simulink model "VDCHyd2020a"  (R2020a)
settings: Solver=daessc  StartTime=0.0  StopTime=simulationEndTime  FixedStep=0.001  RelTol=1e-2
values from neighbouring files (symbols this model uses):
  Bc1_V = [0;0;0;0;0;0]    [initializeSimulationGP.m]
  filtDV = init2ndOrderLowPassFilter(35*2*pi,1,controller.dT)    [initializeLowPassFilters.m]
  filtEnc = init2ndOrderLowPassFilter(35*2*pi,1,controller.dT)    [initializeLowPassFilters.m]
undefined symbols (not defined in the file or in its folder): aux, B11_r_B11Tc1, B11_V, B11_Vr, B11Ftot_r, B12_r_B12Tc2, B12_Rot_Tc2, B12_U_Tc2, B12_V, B12_Vr, B12Ftot_r, B31_r_B31B41, B31_V, B31_Vr, B31FTot_r, B32_r_B32B42, B32_Rot_B42, B32_U_B42, B32_V, B32_Vr, B32FTot_r, B41_r_B41Tc1, B41_V, B41_Vr, B41FTot_r, B42_r_B42Tc2, B42_Rot_Tc2, B42_U_Tc2, B42_V, B42_Vr, B42FTot_r, B52_r_B52P32, B52_Rot_P32, B52_U_P32, B52_V, B52_Vr, B52Ftot_r, Bc1_r_Bc1B11, Bc1_r_Bc1B31, Bc1_Vr, Bc1FTot_r, Bc2_r_Bc2B12, Bc2_r_Bc2B32, Bc2_Rot_B12, Bc2_Rot_B32, Bc2_U_B12, Bc2_U_B32, Bc2_V, Bc2_Vr, Bc2Tot_r, controller, cyl1, cyl2, cylT2, D22_V, D22_Vr, D22Fr, DiscIntNeverNeededParam, dq1, dq11 ... (+125)
libraries: sm_lib x34, nesl_utility x15, simulink x11, dspinverses x1
(part 7 of 12)

== system VDCHyd2020a/sbVDCController/sbFormTotalRequiredForces/sbTotalRequiredForcesPS2/sbProjectionFunctionB52 ==
  note: dP_{B_{52}} / dt = \rho_{B_{52}} s_{B_{52}} \kappa
  sB52 : Inport  PortDimensions=13
  updateActive : Inport  Port=2
  updateReset : Inport  Port=3  PortDimensions=1
  Constant : Constant  Value=update.thetaB52rNominal
  Switch : Switch  Criteria=u2 > Threshold
  discreteIntegratorB52 : DiscreteIntegrator  IntegratorMethod=Integration: Trapezoidal  gainval=update.rhoB52  ExternalReset=level  InitialConditionSource=external  InitialCondition=update.thetaB52rNominal  SampleTime=controller.dT  LimitOutput=on  UpperSaturationLimit=update.thetaB52rUpperBound  LowerSaturationLimit=update.thetaB52rLowerBound  ICPrevOutput=DiscIntNeverNeededParam  ICPrevScaledInput=DiscIntNeverNeededParam
  thetaB52r : Outport
  wires:
  sB52/1 -> discreteIntegratorB52/1  "sB52"
  updateActive/1 -> Switch/2  "updParams"
  Switch/1 -> thetaB52r/1  "thetaB52r"
  Constant/1 -> Switch/3, discreteIntegratorB52/3  "thetaB52rNominal"
  discreteIntegratorB52/1 -> Switch/1  "thetaB52rUpdated"
  updateReset/1 -> discreteIntegratorB52/2  "updateReset"

== system VDCHyd2020a/sbVDCController/sbFormTotalRequiredForces/sbTotalRequiredForcesPS2/sbProjectionFunctionP22 ==
  note: dP_{P_{22}} / dt = \rho_{P_{22}} s_{P_{22}} \kappa
  sP22 : Inport  PortDimensions=13
  updateActive : Inport  Port=2
  updateReset : Inport  Port=3  PortDimensions=1
  Constant : Constant  Value=update.thetaP22rNominal
  Switch : Switch  Criteria=u2 > Threshold
  discreteIntegratorP22 : DiscreteIntegrator  IntegratorMethod=Integration: Trapezoidal  gainval=update.rhoP22  ExternalReset=level  InitialConditionSource=external  InitialCondition=update.thetaP22rNominal  SampleTime=controller.dT  LimitOutput=on  UpperSaturationLimit=update.thetaP22rUpperBound  LowerSaturationLimit=update.thetaP22rLowerBound  ICPrevOutput=DiscIntNeverNeededParam  ICPrevScaledInput=DiscIntNeverNeededParam
  thetaP22r : Outport
  wires:
  updateReset/1 -> discreteIntegratorP22/2  "updateReset"
  discreteIntegratorP22/1 -> Switch/1  "thetaP22rUpdated"
  Constant/1 -> Switch/3, discreteIntegratorP22/3  "thetaP22rNominal"
  Switch/1 -> thetaP22r/1  "thetaP22r"
  updateActive/1 -> Switch/2  "updateActive"
  sP22/1 -> discreteIntegratorP22/1  "sP22"

== system VDCHyd2020a/sbVDCController/sbFormTotalRequiredForces/sbTotalRequiredForcesPS2/sbProjectionFunctionP32 ==
  note: dP_{P_{32}} / dt = \rho_{P_{32}} s_{P_{32}} \kappa
  sP32 : Inport  PortDimensions=13
  updateActive : Inport  Port=2
  updateReset : Inport  Port=3  PortDimensions=1
  Constant : Constant  Value=update.thetaP32rNominal
  Switch : Switch  Criteria=u2 > Threshold
  discreteIntegratorP32 : DiscreteIntegrator  IntegratorMethod=Integration: Trapezoidal  gainval=update.rhoP32  ExternalReset=level  InitialConditionSource=external  InitialCondition=update.thetaP32rNominal  SampleTime=controller.dT  LimitOutput=on  UpperSaturationLimit=update.thetaP32rUpperBound  LowerSaturationLimit=update.thetaP32rLowerBound  ICPrevOutput=DiscIntNeverNeededParam  ICPrevScaledInput=DiscIntNeverNeededParam
  thetaP32r : Outport
  wires:
  updateReset/1 -> discreteIntegratorP32/2  "updateReset"
  discreteIntegratorP32/1 -> Switch/1  "thetaP32rUpdate"
  Constant/1 -> Switch/3, discreteIntegratorP32/3  "thetaP32rNominal"
  Switch/1 -> thetaP32r/1  "thetaP32r"
  updateActive/1 -> Switch/2  "updateActive"
  sP32/1 -> discreteIntegratorP32/1  "sP32"

== system VDCHyd2020a/sbVDCController/sbFormTotalRequiredForces/sbTotalRequiredForcesRS1/sbFilteredVelocityDerivativeB11 ==
  u : Inport
  Demux : Demux  Outputs=6
  Mux : Mux  Inputs=6
  sbDiscreteDerivative1 : Subsystem
  sbDiscreteDerivative2 : Subsystem
  sbDiscreteDerivative3 : Subsystem
  sbDiscreteDerivative4 : Subsystem
  sbDiscreteDerivative5 : Subsystem
  sbDiscreteDerivative6 : Subsystem
  sbLowPassFilter1 : Subsystem
  sbLowPassFilter2 : Subsystem
  sbLowPassFilter3 : Subsystem
  sbLowPassFilter4 : Subsystem
  sbLowPassFilter5 : Subsystem
  sbLowPassFilter6 : Subsystem
  du : Outport
  wires:
  sbLowPassFilter5/1(dVFilt) -> Mux/5
  sbDiscreteDerivative4/1(du/dt) -> sbLowPassFilter4/1(dV)
  sbLowPassFilter4/1(dVFilt) -> Mux/4
  sbLowPassFilter3/1(dVFilt) -> Mux/3
  sbDiscreteDerivative3/1(du/dt) -> sbLowPassFilter3/1(dV)
  sbDiscreteDerivative2/1(du/dt) -> sbLowPassFilter2/1(dV)
  sbLowPassFilter6/1(dVFilt) -> Mux/6
  sbDiscreteDerivative6/1(du/dt) -> sbLowPassFilter6/1(dV)
  sbLowPassFilter1/1(dVFilt) -> Mux/1
  u/1 -> Demux/1
  Demux/2 -> sbDiscreteDerivative2/1(u)
  Demux/5 -> sbDiscreteDerivative5/1(u)
  sbDiscreteDerivative1/1(du/dt) -> sbLowPassFilter1/1(dV)
  Demux/6 -> sbDiscreteDerivative6/1(u)
  sbLowPassFilter2/1(dVFilt) -> Mux/2
  Demux/1 -> sbDiscreteDerivative1/1(u)
  Demux/4 -> sbDiscreteDerivative4/1(u)
  Mux/1 -> du/1
  sbDiscreteDerivative5/1(du/dt) -> sbLowPassFilter5/1(dV)
  Demux/3 -> sbDiscreteDerivative3/1(u)

== system VDCHyd2020a/sbVDCController/sbFormTotalRequiredForces/sbTotalRequiredForcesRS1/sbFilteredVelocityDerivativeB31 ==
  u : Inport
  Demux : Demux  Outputs=6
  Mux : Mux  Inputs=6
  sbDiscreteDerivative1 : Subsystem
  sbDiscreteDerivative2 : Subsystem
  sbDiscreteDerivative3 : Subsystem
  sbDiscreteDerivative4 : Subsystem
  sbDiscreteDerivative5 : Subsystem
  sbDiscreteDerivative6 : Subsystem
  sbLowPassFilter1 : Subsystem
  sbLowPassFilter2 : Subsystem
  sbLowPassFilter3 : Subsystem
  sbLowPassFilter4 : Subsystem
  sbLowPassFilter5 : Subsystem
  sbLowPassFilter6 : Subsystem
  du : Outport
  wires:
  Demux/3 -> sbDiscreteDerivative3/1(u)
  sbDiscreteDerivative5/1(du/dt) -> sbLowPassFilter5/1(dV)
  Mux/1 -> du/1
  Demux/4 -> sbDiscreteDerivative4/1(u)
  Demux/1 -> sbDiscreteDerivative1/1(u)
  sbLowPassFilter2/1(dVFilt) -> Mux/2
  Demux/6 -> sbDiscreteDerivative6/1(u)
  sbDiscreteDerivative1/1(du/dt) -> sbLowPassFilter1/1(dV)
  Demux/5 -> sbDiscreteDerivative5/1(u)
  Demux/2 -> sbDiscreteDerivative2/1(u)
  u/1 -> Demux/1
  sbLowPassFilter1/1(dVFilt) -> Mux/1
  sbDiscreteDerivative6/1(du/dt) -> sbLowPassFilter6/1(dV)
  sbLowPassFilter6/1(dVFilt) -> Mux/6
  sbDiscreteDerivative2/1(du/dt) -> sbLowPassFilter2/1(dV)
  sbDiscreteDerivative3/1(du/dt) -> sbLowPassFilter3/1(dV)
  sbLowPassFilter3/1(dVFilt) -> Mux/3
  sbLowPassFilter4/1(dVFilt) -> Mux/4
  sbDiscreteDerivative4/1(du/dt) -> sbLowPassFilter4/1(dV)
  sbLowPassFilter5/1(dVFilt) -> Mux/5

== system VDCHyd2020a/sbVDCController/sbFormTotalRequiredForces/sbTotalRequiredForcesRS1/sbFilteredVelocityDerivativeB41 ==
  u : Inport
  Demux : Demux  Outputs=6
  Mux : Mux  Inputs=6
  sbDiscreteDerivative1 : Subsystem
  sbDiscreteDerivative2 : Subsystem
  sbDiscreteDerivative3 : Subsystem
  sbDiscreteDerivative4 : Subsystem
  sbDiscreteDerivative5 : Subsystem
  sbDiscreteDerivative6 : Subsystem
  sbLowPassFilter1 : Subsystem
  sbLowPassFilter2 : Subsystem
  sbLowPassFilter3 : Subsystem
  sbLowPassFilter4 : Subsystem
  sbLowPassFilter5 : Subsystem
  sbLowPassFilter6 : Subsystem
  du : Outport
  wires:
  Demux/3 -> sbDiscreteDerivative3/1(u)
  sbDiscreteDerivative5/1(du/dt) -> sbLowPassFilter5/1(dV)
  Mux/1 -> du/1
  Demux/4 -> sbDiscreteDerivative4/1(u)
  Demux/1 -> sbDiscreteDerivative1/1(u)
  sbLowPassFilter2/1(dVFilt) -> Mux/2
  Demux/6 -> sbDiscreteDerivative6/1(u)
  sbDiscreteDerivative1/1(du/dt) -> sbLowPassFilter1/1(dV)
  Demux/5 -> sbDiscreteDerivative5/1(u)
  Demux/2 -> sbDiscreteDerivative2/1(u)
  u/1 -> Demux/1
  sbLowPassFilter1/1(dVFilt) -> Mux/1
  sbDiscreteDerivative6/1(du/dt) -> sbLowPassFilter6/1(dV)
  sbLowPassFilter6/1(dVFilt) -> Mux/6
  sbDiscreteDerivative2/1(du/dt) -> sbLowPassFilter2/1(dV)
  sbDiscreteDerivative3/1(du/dt) -> sbLowPassFilter3/1(dV)
  sbLowPassFilter3/1(dVFilt) -> Mux/3
  sbLowPassFilter4/1(dVFilt) -> Mux/4
  sbDiscreteDerivative4/1(du/dt) -> sbLowPassFilter4/1(dV)
  sbLowPassFilter5/1(dVFilt) -> Mux/5

== system VDCHyd2020a/sbVDCController/sbFormTotalRequiredForces/sbTotalRequiredForcesRS1/sbFilteredVelocityDerivativeBc1 ==
  u : Inport
  Demux : Demux  Outputs=6
  Mux : Mux  Inputs=6
  sbDiscreteDerivative1 : Subsystem
  sbDiscreteDerivative2 : Subsystem
  sbDiscreteDerivative3 : Subsystem
  sbDiscreteDerivative4 : Subsystem
  sbDiscreteDerivative5 : Subsystem
  sbDiscreteDerivative6 : Subsystem
  sbLowPassFilter1 : Subsystem
  sbLowPassFilter2 : Subsystem
  sbLowPassFilter3 : Subsystem
  sbLowPassFilter4 : Subsystem
  sbLowPassFilter5 : Subsystem
  sbLowPassFilter6 : Subsystem
  du : Outport
  wires:
  sbLowPassFilter5/1(dVFilt) -> Mux/5
  sbDiscreteDerivative4/1(du/dt) -> sbLowPassFilter4/1(dV)
  sbLowPassFilter4/1(dVFilt) -> Mux/4
  sbLowPassFilter3/1(dVFilt) -> Mux/3
  sbDiscreteDerivative3/1(du/dt) -> sbLowPassFilter3/1(dV)
  sbDiscreteDerivative2/1(du/dt) -> sbLowPassFilter2/1(dV)
  sbLowPassFilter6/1(dVFilt) -> Mux/6
  sbDiscreteDerivative6/1(du/dt) -> sbLowPassFilter6/1(dV)
  sbLowPassFilter1/1(dVFilt) -> Mux/1
  u/1 -> Demux/1
  Demux/2 -> sbDiscreteDerivative2/1(u)
  Demux/5 -> sbDiscreteDerivative5/1(u)
  sbDiscreteDerivative1/1(du/dt) -> sbLowPassFilter1/1(dV)
  Demux/6 -> sbDiscreteDerivative6/1(u)
  sbLowPassFilter2/1(dVFilt) -> Mux/2
  Demux/1 -> sbDiscreteDerivative1/1(u)
  Demux/4 -> sbDiscreteDerivative4/1(u)
  Mux/1 -> du/1
  sbDiscreteDerivative5/1(du/dt) -> sbLowPassFilter5/1(dV)
  Demux/3 -> sbDiscreteDerivative3/1(u)

== system VDCHyd2020a/sbVDCController/sbFormTotalRequiredForces/sbTotalRequiredForcesRS1/sbProjectionFunctionB11 ==
  note: dP_{B_{11}} / dt = \rho_{B_{11}} s_{B_{11}} \kappa
  sB11 : Inport  PortDimensions=13
  updateActive : Inport  Port=2
  updateReset : Inport  Port=3  PortDimensions=1
  Constant : Constant  Value=update.thetaB11rNominal
  Switch : Switch  Criteria=u2 > Threshold
  discreteIntegratorPB11 : DiscreteIntegrator  IntegratorMethod=Integration: Trapezoidal  gainval=update.rhoB11  ExternalReset=level  InitialConditionSource=external  InitialCondition=update.thetaB11rNominal  SampleTime=controller.dT  LimitOutput=on  UpperSaturationLimit=update.thetaB11rUpperBound  LowerSaturationLimit=update.thetaB11rLowerBound  ICPrevOutput=DiscIntNeverNeededParam  ICPrevScaledInput=DiscIntNeverNeededParam
  thetaB11r : Outport
  wires:
  sB11/1 -> discreteIntegratorPB11/1  "sB11"
  updateActive/1 -> Switch/2
  Switch/1 -> thetaB11r/1  "thetaB11r"
  Constant/1 -> Switch/3, discreteIntegratorPB11/3  "thetaB11rNominal"
  discreteIntegratorPB11/1 -> Switch/1  "thetaB11rUpdated"
  updateReset/1 -> discreteIntegratorPB11/2  "updateReset"

== system VDCHyd2020a/sbVDCController/sbFormTotalRequiredForces/sbTotalRequiredForcesRS1/sbProjectionFunctionB31 ==
  note: dP_{B_{31}} / dt = \rho_{B_{31}} s_{B_{31}} \kappa
  sB31 : Inport  PortDimensions=13
  updateActive : Inport  Port=2
  updateReset : Inport  Port=3  PortDimensions=1
  Constant : Constant  Value=update.thetaB31rNominal
  Switch : Switch  Criteria=u2 > Threshold
  discreteIntegratorB31 : DiscreteIntegrator  IntegratorMethod=Integration: Trapezoidal  gainval=update.rhoB31  ExternalReset=level  InitialConditionSource=external  InitialCondition=update.thetaB31rNominal  SampleTime=controller.dT  LimitOutput=on  UpperSaturationLimit=update.thetaB31rUpperBound  LowerSaturationLimit=update.thetaB31rLowerBound  ICPrevOutput=DiscIntNeverNeededParam  ICPrevScaledInput=DiscIntNeverNeededParam
  thetaB31r : Outport
  wires:
  updateReset/1 -> discreteIntegratorB31/2  "updateReset"
  discreteIntegratorB31/1 -> Switch/1  "thetaB31rUpdated"
  Constant/1 -> Switch/3, discreteIntegratorB31/3  "thetaB31rNominal"
  Switch/1 -> thetaB31r/1  "thetaB31r"
  updateActive/1 -> Switch/2  "updateActive"
  sB31/1 -> discreteIntegratorB31/1  "sB31"

== system VDCHyd2020a/sbVDCController/sbFormTotalRequiredForces/sbTotalRequiredForcesRS1/sbProjectionFunctionB41 ==
  note: dP_{B_{41}} / dt = \rho_{B_{41}} s_{B_{41}} \kappa
  sB41 : Inport  PortDimensions=13
  updateActive : Inport  Port=2
  updateReset : Inport  Port=3  PortDimensions=1
  Constant : Constant  Value=update.thetaB41rNominal
  Discrete-Time Integrator1 : DiscreteIntegrator  IntegratorMethod=Integration: Trapezoidal  gainval=update.rhoB41  ExternalReset=level  InitialConditionSource=external  InitialCondition=update.thetaB41rNominal  SampleTime=controller.dT  LimitOutput=on  UpperSaturationLimit=update.thetaB41rUpperBound  LowerSaturationLimit=update.thetaB41rLowerBound  ICPrevOutput=DiscIntNeverNeededParam  ICPrevScaledInput=DiscIntNeverNeededParam
  Switch : Switch  Criteria=u2 > Threshold
  thetaB41r : Outport
  wires:
  sB41/1 -> Discrete-Time Integrator1/1  "sB41"
  updateActive/1 -> Switch/2  "updateActive"
  Switch/1 -> thetaB41r/1  "thetaB41r"
  Constant/1 -> Switch/3, Discrete-Time Integrator1/3  "thetaB41rNominal"
  Discrete-Time Integrator1/1 -> Switch/1  "thetaB41rUpdated"
  updateReset/1 -> Discrete-Time Integrator1/2  "updateReset"

== system VDCHyd2020a/sbVDCController/sbFormTotalRequiredForces/sbTotalRequiredForcesRS1/sbProjectionFunctionBc1 ==
  note: dP_{B_{c1}} / dt = \rho_{B_{c1}} s_{B_{c1}} \kappa
  sBc1 : Inport  PortDimensions=13
  updateActive : Inport  Port=2
  updateReset : Inport  Port=3  PortDimensions=1
  Constant : Constant  Value=update.thetaBc1rNominal
  Switch : Switch  Criteria=u2 > Threshold
  discreteIntegratorPBc1 : DiscreteIntegrator  IntegratorMethod=Integration: Trapezoidal  gainval=update.rhoBc1  ExternalReset=level  InitialConditionSource=external  InitialCondition=update.thetaBc1rNominal  SampleTime=controller.dT  LimitOutput=on  UpperSaturationLimit=update.thetaBc1rUpperBound  LowerSaturationLimit=update.thetaBc1rLowerBound  ICPrevOutput=DiscIntNeverNeededParam  ICPrevScaledInput=DiscIntNeverNeededParam
  thetaBc1r : Outport
  wires:
  discreteIntegratorPBc1/1 -> Switch/1  "thetaBc1rUpdated"
  Constant/1 -> Switch/3, discreteIntegratorPBc1/3  "thetaBc1rNominal"
  Switch/1 -> thetaBc1r/1  "thetaBc1r"
  updateActive/1 -> Switch/2  "updateActive"
  sBc1/1 -> discreteIntegratorPBc1/1  "sBc1"
  updateReset/1 -> discreteIntegratorPBc1/2  "updateReset"

== system VDCHyd2020a/sbVDCController/sbFormTotalRequiredForces/sbTotalRequiredForcesRS2/sbFilteredVelocityDerivativeB12 ==
  u : Inport
  Demux : Demux  Outputs=6
  Mux : Mux  Inputs=6
  sbDiscreteDerivative1 : Subsystem
  sbDiscreteDerivative2 : Subsystem
  sbDiscreteDerivative3 : Subsystem
  sbDiscreteDerivative4 : Subsystem
  sbDiscreteDerivative5 : Subsystem
  sbDiscreteDerivative6 : Subsystem
  sbLowPassFilter1 : Subsystem
  sbLowPassFilter2 : Subsystem
  sbLowPassFilter3 : Subsystem
  sbLowPassFilter4 : Subsystem
  sbLowPassFilter5 : Subsystem
  sbLowPassFilter6 : Subsystem
  du : Outport
  wires:
  Demux/3 -> sbDiscreteDerivative3/1(u)
  sbDiscreteDerivative5/1(du/dt) -> sbLowPassFilter5/1(dV)
  Mux/1 -> du/1
  Demux/4 -> sbDiscreteDerivative4/1(u)
  Demux/1 -> sbDiscreteDerivative1/1(u)
  sbLowPassFilter2/1(dVFilt) -> Mux/2
  Demux/6 -> sbDiscreteDerivative6/1(u)
  sbDiscreteDerivative1/1(du/dt) -> sbLowPassFilter1/1(dV)
  Demux/5 -> sbDiscreteDerivative5/1(u)
  Demux/2 -> sbDiscreteDerivative2/1(u)
  u/1 -> Demux/1
  sbLowPassFilter1/1(dVFilt) -> Mux/1
  sbDiscreteDerivative6/1(du/dt) -> sbLowPassFilter6/1(dV)
  sbLowPassFilter6/1(dVFilt) -> Mux/6
  sbDiscreteDerivative2/1(du/dt) -> sbLowPassFilter2/1(dV)
  sbDiscreteDerivative3/1(du/dt) -> sbLowPassFilter3/1(dV)
  sbLowPassFilter3/1(dVFilt) -> Mux/3
  sbLowPassFilter4/1(dVFilt) -> Mux/4
  sbDiscreteDerivative4/1(du/dt) -> sbLowPassFilter4/1(dV)
  sbLowPassFilter5/1(dVFilt) -> Mux/5

== system VDCHyd2020a/sbVDCController/sbFormTotalRequiredForces/sbTotalRequiredForcesRS2/sbFilteredVelocityDerivativeB32 ==
  u : Inport
  Demux : Demux  Outputs=6
  Mux : Mux  Inputs=6
  sbDiscreteDerivative1 : Subsystem
  sbDiscreteDerivative2 : Subsystem
  sbDiscreteDerivative3 : Subsystem
  sbDiscreteDerivative4 : Subsystem
  sbDiscreteDerivative5 : Subsystem
  sbDiscreteDerivative6 : Subsystem
  sbLowPassFilter1 : Subsystem
  sbLowPassFilter2 : Subsystem
  sbLowPassFilter3 : Subsystem
  sbLowPassFilter4 : Subsystem
  sbLowPassFilter5 : Subsystem
  sbLowPassFilter6 : Subsystem
  du : Outport
  wires:
  Demux/3 -> sbDiscreteDerivative3/1(u)
  sbDiscreteDerivative5/1(du/dt) -> sbLowPassFilter5/1(dV)
  Mux/1 -> du/1
  Demux/4 -> sbDiscreteDerivative4/1(u)
  Demux/1 -> sbDiscreteDerivative1/1(u)
  sbLowPassFilter2/1(dVFilt) -> Mux/2
  Demux/6 -> sbDiscreteDerivative6/1(u)
  sbDiscreteDerivative1/1(du/dt) -> sbLowPassFilter1/1(dV)
  Demux/5 -> sbDiscreteDerivative5/1(u)
  Demux/2 -> sbDiscreteDerivative2/1(u)
  u/1 -> Demux/1
  sbLowPassFilter1/1(dVFilt) -> Mux/1
  sbDiscreteDerivative6/1(du/dt) -> sbLowPassFilter6/1(dV)
  sbLowPassFilter6/1(dVFilt) -> Mux/6
  sbDiscreteDerivative2/1(du/dt) -> sbLowPassFilter2/1(dV)
  sbDiscreteDerivative3/1(du/dt) -> sbLowPassFilter3/1(dV)
  sbLowPassFilter3/1(dVFilt) -> Mux/3
  sbLowPassFilter4/1(dVFilt) -> Mux/4
  sbDiscreteDerivative4/1(du/dt) -> sbLowPassFilter4/1(dV)
  sbLowPassFilter5/1(dVFilt) -> Mux/5

== system VDCHyd2020a/sbVDCController/sbFormTotalRequiredForces/sbTotalRequiredForcesRS2/sbFilteredVelocityDerivativeB42 ==
  u : Inport
  Demux : Demux  Outputs=6
  Mux : Mux  Inputs=6
  sbDiscreteDerivative1 : Subsystem
  sbDiscreteDerivative2 : Subsystem
  sbDiscreteDerivative3 : Subsystem
  sbDiscreteDerivative4 : Subsystem
  sbDiscreteDerivative5 : Subsystem
  sbDiscreteDerivative6 : Subsystem
  sbLowPassFilter1 : Subsystem
  sbLowPassFilter2 : Subsystem
  sbLowPassFilter3 : Subsystem
  sbLowPassFilter4 : Subsystem
  sbLowPassFilter5 : Subsystem
  sbLowPassFilter6 : Subsystem
  du : Outport
  wires:
  Demux/3 -> sbDiscreteDerivative3/1(u)
  sbDiscreteDerivative5/1(du/dt) -> sbLowPassFilter5/1(dV)
  Mux/1 -> du/1
  Demux/4 -> sbDiscreteDerivative4/1(u)
  Demux/1 -> sbDiscreteDerivative1/1(u)
  sbLowPassFilter2/1(dVFilt) -> Mux/2
  Demux/6 -> sbDiscreteDerivative6/1(u)
  sbDiscreteDerivative1/1(du/dt) -> sbLowPassFilter1/1(dV)
  Demux/5 -> sbDiscreteDerivative5/1(u)
  Demux/2 -> sbDiscreteDerivative2/1(u)
  u/1 -> Demux/1
  sbLowPassFilter1/1(dVFilt) -> Mux/1
  sbDiscreteDerivative6/1(du/dt) -> sbLowPassFilter6/1(dV)
  sbLowPassFilter6/1(dVFilt) -> Mux/6
  sbDiscreteDerivative2/1(du/dt) -> sbLowPassFilter2/1(dV)
  sbDiscreteDerivative3/1(du/dt) -> sbLowPassFilter3/1(dV)
  sbLowPassFilter3/1(dVFilt) -> Mux/3
  sbLowPassFilter4/1(dVFilt) -> Mux/4
  sbDiscreteDerivative4/1(du/dt) -> sbLowPassFilter4/1(dV)
  sbLowPassFilter5/1(dVFilt) -> Mux/5

== system VDCHyd2020a/sbVDCController/sbFormTotalRequiredForces/sbTotalRequiredForcesRS2/sbFilteredVelocityDerivativeBc2 ==
  u : Inport
  Demux : Demux  Outputs=6
  Mux : Mux  Inputs=6
  sbDiscreteDerivative1 : Subsystem
  sbDiscreteDerivative2 : Subsystem
  sbDiscreteDerivative3 : Subsystem
  sbDiscreteDerivative4 : Subsystem
  sbDiscreteDerivative5 : Subsystem
  sbDiscreteDerivative6 : Subsystem
  sbLowPassFilter1 : Subsystem
  sbLowPassFilter2 : Subsystem
  sbLowPassFilter3 : Subsystem
  sbLowPassFilter4 : Subsystem
  sbLowPassFilter5 : Subsystem
  sbLowPassFilter6 : Subsystem
  du : Outport
  wires:
  Demux/3 -> sbDiscreteDerivative3/1(u)
  sbDiscreteDerivative5/1(du/dt) -> sbLowPassFilter5/1(dV)
  Mux/1 -> du/1
  Demux/4 -> sbDiscreteDerivative4/1(u)
  Demux/1 -> sbDiscreteDerivative1/1(u)
  sbLowPassFilter2/1(dVFilt) -> Mux/2
  Demux/6 -> sbDiscreteDerivative6/1(u)
  sbDiscreteDerivative1/1(du/dt) -> sbLowPassFilter1/1(dV)
  Demux/5 -> sbDiscreteDerivative5/1(u)
  Demux/2 -> sbDiscreteDerivative2/1(u)
  u/1 -> Demux/1
  sbLowPassFilter1/1(dVFilt) -> Mux/1
  sbDiscreteDerivative6/1(du/dt) -> sbLowPassFilter6/1(dV)
  sbLowPassFilter6/1(dVFilt) -> Mux/6
  sbDiscreteDerivative2/1(du/dt) -> sbLowPassFilter2/1(dV)
  sbDiscreteDerivative3/1(du/dt) -> sbLowPassFilter3/1(dV)
  sbLowPassFilter3/1(dVFilt) -> Mux/3
  sbLowPassFilter4/1(dVFilt) -> Mux/4
  sbDiscreteDerivative4/1(du/dt) -> sbLowPassFilter4/1(dV)
  sbLowPassFilter5/1(dVFilt) -> Mux/5

== system VDCHyd2020a/sbVDCController/sbFormTotalRequiredForces/sbTotalRequiredForcesRS2/sbProjectionFunctionB12 ==
  note: dP_{B_{12}} / dt = \rho_{B_{12}} s_{B_{12}} \kappa
  sB12 : Inport  PortDimensions=13
  updateActive : Inport  Port=2
  updateReset : Inport  Port=3  PortDimensions=1
  Constant : Constant  Value=update.thetaB12rNominal
  Switch : Switch  Criteria=u2 > Threshold
  discreteIntegratorB12 : DiscreteIntegrator  IntegratorMethod=Integration: Trapezoidal  gainval=update.rhoB12  ExternalReset=level  InitialConditionSource=external  InitialCondition=update.thetaB12rNominal  SampleTime=controller.dT  LimitOutput=on  UpperSaturationLimit=update.thetaB12rUpperBound  LowerSaturationLimit=update.thetaB12rLowerBound  ICPrevOutput=DiscIntNeverNeededParam  ICPrevScaledInput=DiscIntNeverNeededParam
  thetaB12r : Outport
  wires:
  updateReset/1 -> discreteIntegratorB12/2  "updateReset"
  discreteIntegratorB12/1 -> Switch/1  "thetaB12rUpdated"
  Constant/1 -> Switch/3, discreteIntegratorB12/3  "thetaB12rNominal"
  Switch/1 -> thetaB12r/1  "thetaB12r"
  updateActive/1 -> Switch/2  "updateActive"
  sB12/1 -> discreteIntegratorB12/1  "sB12"

== system VDCHyd2020a/sbVDCController/sbFormTotalRequiredForces/sbTotalRequiredForcesRS2/sbProjectionFunctionB32 ==
  note: dP_{B_{32}} / dt = \rho_{B_{32}} s_{B_{32}} \kappa
  sB32 : Inport  PortDimensions=13
  updateActive : Inport  Port=2
  updateReset : Inport  Port=3  PortDimensions=1
  Constant : Constant  Value=update.thetaB32rNominal
  Switch : Switch  Criteria=u2 > Threshold
  discreteIntegratorB32 : DiscreteIntegrator  IntegratorMethod=Integration: Trapezoidal  gainval=update.rhoB32  ExternalReset=level  InitialConditionSource=external  InitialCondition=update.thetaB32rNominal  SampleTime=controller.dT  LimitOutput=on  UpperSaturationLimit=update.thetaB32rUpperBound  LowerSaturationLimit=update.thetaB32rLowerBound  ICPrevOutput=DiscIntNeverNeededParam  ICPrevScaledInput=DiscIntNeverNeededParam
  thetaB32r : Outport
  wires:
  sB32/1 -> discreteIntegratorB32/1  "sB32"
  updateActive/1 -> Switch/2  "updateActive"
  Switch/1 -> thetaB32r/1  "thetaB32r"
  Constant/1 -> Switch/3, discreteIntegratorB32/3  "thetaB32rNominal"
  discreteIntegratorB32/1 -> Switch/1  "thetaB32rUpdated"
  updateReset/1 -> discreteIntegratorB32/2  "updateReset"

== system VDCHyd2020a/sbVDCController/sbFormTotalRequiredForces/sbTotalRequiredForcesRS2/sbProjectionFunctionB42 ==
  note: dP_{B_{42}} / dt = \rho_{B_{42}} s_{B_{42}} \kappa
  sB42 : Inport  PortDimensions=13
  updateActive : Inport  Port=2
  updateReset : Inport  Port=3  PortDimensions=1
  Constant : Constant  Value=update.thetaB42rNominal
  Switch : Switch  Criteria=u2 > Threshold
  discreteIntegratorB42 : DiscreteIntegrator  IntegratorMethod=Integration: Trapezoidal  gainval=update.rhoB42  ExternalReset=level  InitialConditionSource=external  InitialCondition=update.thetaB42rNominal  SampleTime=controller.dT  LimitOutput=on  UpperSaturationLimit=update.thetaB42rUpperBound  LowerSaturationLimit=update.thetaB42rLowerBound  ICPrevOutput=DiscIntNeverNeededParam  ICPrevScaledInput=DiscIntNeverNeededParam
  thetaB42r : Outport
  wires:
  updateReset/1 -> discreteIntegratorB42/2  "updateReset"
  discreteIntegratorB42/1 -> Switch/1  "thetaB42rUpdated"
  Constant/1 -> Switch/3, discreteIntegratorB42/3  "thetaB42rNominal"
  Switch/1 -> thetaB42r/1  "thetaB42r"
  updateActive/1 -> Switch/2  "updateActive"
  sB42/1 -> discreteIntegratorB42/1  "sB42"

== system VDCHyd2020a/sbVDCController/sbFormTotalRequiredForces/sbTotalRequiredForcesRS2/sbProjectionFunctionBc2 ==
  note: dP_{B_{c2}} / dt = \rho_{B_{c2}} s_{B_{c2}} \kappa
  sBc2 : Inport  PortDimensions=13
  updateActive : Inport  Port=2
  updateReset : Inport  Port=3  PortDimensions=1
  Constant : Constant  Value=update.thetaBc2rNominal
  Switch : Switch  Criteria=u2 > Threshold
  discreteIntegratorBc2 : DiscreteIntegrator  IntegratorMethod=Integration: Trapezoidal  gainval=update.rhoBc2  ExternalReset=level  InitialConditionSource=external  InitialCondition=update.thetaBc2rNominal  SampleTime=controller.dT  LimitOutput=on  UpperSaturationLimit=update.thetaBc2rUpperBound  LowerSaturationLimit=update.thetaBc2rLowerBound  ICPrevOutput=DiscIntNeverNeededParam  ICPrevScaledInput=DiscIntNeverNeededParam
  thetaBc2r : Outport
  wires:
  sBc2/1 -> discreteIntegratorBc2/1  "sBc2"
  updateActive/1 -> Switch/2  "updateActive"
  Switch/1 -> thetaBc2r/1  "thetaBc2r"
  Constant/1 -> Switch/3, discreteIntegratorBc2/3  "thetaBc2rNominal"
  discreteIntegratorBc2/1 -> Switch/1  "thetaBc2rUpdated"
  updateReset/1 -> discreteIntegratorBc2/2  "updateReset"

== system VDCHyd2020a/sbVDCController/sbFormingControlActions/sbFrictionRegressorPS2/sbAverageDeformationOfBristlesPS2 ==
  note: z^{'}_j = v_j - |v_j| \cdot z_j/z_{ssj}
  dxt2 : Inport
  Abs : Abs
  Constant : Constant  Value=frictionPS2.zss
  Discrete-Time Integrator : DiscreteIntegrator  SampleTime=controller.dT  ICPrevOutput=DiscIntNeverNeededParam  ICPrevScaledInput=DiscIntNeverNeededParam
  Divide : Product  Inputs=**/
  Sum : Sum  Inputs=|+-
  zt2 : Outport
  wires:
  dxt2/1 -> Sum/1, Abs/1
  Divide/1 -> Sum/2
  Abs/1 -> Divide/1
  Discrete-Time Integrator/1 -> zt2/1, Divide/2
  Constant/1 -> Divide/3
  Sum/1 -> Discrete-Time Integrator/1

== system VDCHyd2020a/sbVDCController/sbFormingControlActions/sbFrictionRegressorPS2/sbFrictionSwitchingFunctionPS2 ==
  dxt2 : Inport
  Abs : Abs
  Constant : Constant  Value=frictionPS2.delta1
  Constant1 : Constant
  Constant2 : Constant
  Discrete-Time Integrator : DiscreteIntegrator  SampleTime=controller.dT  ICPrevOutput=DiscIntNeverNeededParam  ICPrevScaledInput=DiscIntNeverNeededParam
  Divide : Product  Inputs=*/
  Gain : Gain  Gain=10
  Product : Product
  Product1 : Product  Inputs=3
  Sum : Sum  Inputs=|+-
  Sum1 : Sum  Inputs=|++
  LPS2 : Outport
  wires:
  Gain/1 -> Discrete-Time Integrator/1
  Sum/1 -> Gain/1
  Abs/1 -> Sum/1
  dxt2/1 -> Abs/1
  Discrete-Time Integrator/1 -> Product/1, Sum/2
  Constant/1 -> Product/2
  Product/1 -> Product1/1, Product1/3, Product1/2
  Product1/1 -> Sum1/1
  Constant1/1 -> Sum1/2
  Sum1/1 -> Divide/2
  Constant2/1 -> Divide/1
  Divide/1 -> LPS2/1

== system VDCHyd2020a/sbVDCController/sbFormingControlActions/sbFrictionRegressorRS1/sbAverageDeformationOfBristlesRS2 ==
  note: z^{'}_j = v_j - |v_j| \cdot z_j/z_{ssj}
  dx1 : Inport
  Abs : Abs
  Constant : Constant  Value=frictionRS1.zss
  Discrete-Time Integrator : DiscreteIntegrator  SampleTime=controller.dT  ICPrevOutput=DiscIntNeverNeededParam  ICPrevScaledInput=DiscIntNeverNeededParam
  Divide : Product  Inputs=**/
  Sum : Sum  Inputs=|+-
  z1 : Outport
  wires:
  dx1/1 -> Sum/1, Abs/1
  Divide/1 -> Sum/2
  Abs/1 -> Divide/1
  Discrete-Time Integrator/1 -> z1/1, Divide/2
  Constant/1 -> Divide/3
  Sum/1 -> Discrete-Time Integrator/1

== system VDCHyd2020a/sbVDCController/sbFormingControlActions/sbFrictionRegressorRS1/sbFrictionSwitchingFunctionRS2 ==
  dx1 : Inport
  Abs : Abs
  Constant : Constant  Value=frictionRS1.delta1
  Constant1 : Constant
  Constant2 : Constant
  Discrete-Time Integrator : DiscreteIntegrator  SampleTime=controller.dT  ICPrevOutput=DiscIntNeverNeededParam  ICPrevScaledInput=DiscIntNeverNeededParam
  Divide : Product  Inputs=*/
  Gain : Gain  Gain=10
  Product : Product
  Product1 : Product  Inputs=3
  Sum : Sum  Inputs=|+-
  Sum1 : Sum  Inputs=|++
  LRS1 : Outport
  wires:
  Gain/1 -> Discrete-Time Integrator/1
  Sum/1 -> Gain/1
  Abs/1 -> Sum/1
  dx1/1 -> Abs/1
  Discrete-Time Integrator/1 -> Product/1, Sum/2
  Constant/1 -> Product/2
  Product/1 -> Product1/1, Product1/3, Product1/2
  Product1/1 -> Sum1/1
  Constant1/1 -> Sum1/2
  Sum1/1 -> Divide/2
  Constant2/1 -> Divide/1
  Divide/1 -> LRS1/1

== system VDCHyd2020a/sbVDCController/sbFormingControlActions/sbFrictionRegressorRS2/sbAverageDeformationOfBristlesRS2 ==
  note: z^{'}_j = v_j - |v_j| \cdot z_j/z_{ssj}
  dx2 : Inport
  Abs : Abs
  Constant : Constant  Value=frictionRS2.zss
  Discrete-Time Integrator : DiscreteIntegrator  SampleTime=controller.dT  ICPrevOutput=DiscIntNeverNeededParam  ICPrevScaledInput=DiscIntNeverNeededParam
  Divide : Product  Inputs=**/
  Sum : Sum  Inputs=|+-
  z2 : Outport
  wires:
  dx2/1 -> Sum/1, Abs/1
  Divide/1 -> Sum/2
  Abs/1 -> Divide/1
  Discrete-Time Integrator/1 -> z2/1, Divide/2
  Constant/1 -> Divide/3
  Sum/1 -> Discrete-Time Integrator/1

== system VDCHyd2020a/sbVDCController/sbFormingControlActions/sbFrictionRegressorRS2/sbFrictionSwitchingFunctionRS2 ==
  dx2 : Inport
  Abs : Abs
  Constant : Constant  Value=frictionRS2.delta1
  Constant1 : Constant
  Constant2 : Constant
  Discrete-Time Integrator : DiscreteIntegrator  SampleTime=controller.dT  ICPrevOutput=DiscIntNeverNeededParam  ICPrevScaledInput=DiscIntNeverNeededParam
  Divide : Product  Inputs=*/
  Gain : Gain  Gain=10
  Product : Product
  Product1 : Product  Inputs=3
  Sum : Sum  Inputs=|+-
  Sum1 : Sum  Inputs=|++
  LRS2 : Outport
  wires:
  Gain/1 -> Discrete-Time Integrator/1
  Sum/1 -> Gain/1
  Abs/1 -> Sum/1
  dx2/1 -> Abs/1
  Discrete-Time Integrator/1 -> Product/1, Sum/2
  Constant/1 -> Product/2
  Product/1 -> Product1/1, Product1/3, Product1/2
  Product1/1 -> Sum1/1
  Constant1/1 -> Sum1/2
  Sum1/1 -> Divide/2
  Constant2/1 -> Divide/1
  Divide/1 -> LRS2/1

== system VDCHyd2020a/sbHydraulicManipulatorSimscape/sbLiftCylinderAndLiftPiston/sbFrictionForceRS1/sbFrictionRegressorRS1/sbAverageDeformationOfBristlesRS2 ==
  note: z^{'}_j = v_j - |v_j| \cdot z_j/z_{ssj}
  dx1 : Inport
  Abs : Abs
  Constant : Constant  Value=frictionRS1.zss
  Discrete-Time Integrator : DiscreteIntegrator  SampleTime=controller.dT  ICPrevOutput=DiscIntNeverNeededParam  ICPrevScaledInput=DiscIntNeverNeededParam
  Divide : Product  Inputs=**/
  Sum : Sum  Inputs=|+-
  z1 : Outport
  wires:
  dx1/1 -> Sum/1, Abs/1
  Divide/1 -> Sum/2
  Abs/1 -> Divide/1
  Discrete-Time Integrator/1 -> z1/1, Divide/2
  Constant/1 -> Divide/3
  Sum/1 -> Discrete-Time Integrator/1

== system VDCHyd2020a/sbHydraulicManipulatorSimscape/sbLiftCylinderAndLiftPiston/sbFrictionForceRS1/sbFrictionRegressorRS1/sbFrictionSwitchingFunctionRS2 ==
  dx1 : Inport
  Abs : Abs
  Constant : Constant  Value=frictionRS1.delta1
  Constant1 : Constant
  Constant2 : Constant
  Discrete-Time Integrator : DiscreteIntegrator  SampleTime=controller.dT  ICPrevOutput=DiscIntNeverNeededParam  ICPrevScaledInput=DiscIntNeverNeededParam
  Divide : Product  Inputs=*/
  Gain : Gain  Gain=10
  Product : Product
  Product1 : Product  Inputs=3
  Sum : Sum  Inputs=|+-
  Sum1 : Sum  Inputs=|++
  LRS1 : Outport
  wires:
  Gain/1 -> Discrete-Time Integrator/1
  Sum/1 -> Gain/1
  Abs/1 -> Sum/1
  dx1/1 -> Abs/1
  Discrete-Time Integrator/1 -> Product/1, Sum/2
  Constant/1 -> Product/2
  Product/1 -> Product1/1, Product1/3, Product1/2
  Product1/1 -> Sum1/1
  Constant1/1 -> Sum1/2
  Sum1/1 -> Divide/2
  Constant2/1 -> Divide/1
  Divide/1 -> LRS1/1

== system VDCHyd2020a/sbHydraulicManipulatorSimscape/sbPrismaticJointCylinderAndPiston/sbFrictionForcePS2/sbFrictionRegressorPS2/sbAverageDeformationOfBristlesPS2 ==
  note: z^{'}_j = v_j - |v_j| \cdot z_j/z_{ssj}
  dxt2 : Inport
  Abs : Abs
  Constant : Constant  Value=frictionPS2.zss
  Discrete-Time Integrator : DiscreteIntegrator  SampleTime=controller.dT  ICPrevOutput=DiscIntNeverNeededParam  ICPrevScaledInput=DiscIntNeverNeededParam
  Divide : Product  Inputs=**/
  Sum : Sum  Inputs=|+-
  zt2 : Outport
  wires:
  dxt2/1 -> Sum/1, Abs/1
  Divide/1 -> Sum/2
  Abs/1 -> Divide/1
  Discrete-Time Integrator/1 -> zt2/1, Divide/2
  Constant/1 -> Divide/3
  Sum/1 -> Discrete-Time Integrator/1

== system VDCHyd2020a/sbHydraulicManipulatorSimscape/sbPrismaticJointCylinderAndPiston/sbFrictionForcePS2/sbFrictionRegressorPS2/sbFrictionSwitchingFunctionPS2 ==
  dxt2 : Inport
  Abs : Abs
  Constant : Constant  Value=frictionPS2.delta1
  Constant1 : Constant
  Constant2 : Constant
  Discrete-Time Integrator : DiscreteIntegrator  SampleTime=controller.dT  ICPrevOutput=DiscIntNeverNeededParam  ICPrevScaledInput=DiscIntNeverNeededParam
  Divide : Product  Inputs=*/
  Gain : Gain  Gain=10
  Product : Product
  Product1 : Product  Inputs=3
  Sum : Sum  Inputs=|+-
  Sum1 : Sum  Inputs=|++
  LPS2 : Outport
  wires:
  Gain/1 -> Discrete-Time Integrator/1
  Sum/1 -> Gain/1
  Abs/1 -> Sum/1
  dxt2/1 -> Abs/1
  Discrete-Time Integrator/1 -> Product/1, Sum/2
  Constant/1 -> Product/2
  Product/1 -> Product1/1, Product1/3, Product1/2
  Product1/1 -> Sum1/1
  Constant1/1 -> Sum1/2
  Sum1/1 -> Divide/2
  Constant2/1 -> Divide/1
  Divide/1 -> LPS2/1

== system VDCHyd2020a/sbHydraulicManipulatorSimscape/sbTiltCylinderAndTiltPiston/sbFrictionForceRS2/sbFrictionRegressorRS2/sbAverageDeformationOfBristlesRS2 ==
  note: z^{'}_j = v_j - |v_j| \cdot z_j/z_{ssj}
  dx2 : Inport
  Abs : Abs
  Constant : Constant  Value=frictionRS2.zss
  Discrete-Time Integrator : DiscreteIntegrator  SampleTime=controller.dT  ICPrevOutput=DiscIntNeverNeededParam  ICPrevScaledInput=DiscIntNeverNeededParam
  Divide : Product  Inputs=**/
  Sum : Sum  Inputs=|+-
  z2 : Outport
  wires:
  dx2/1 -> Sum/1, Abs/1
  Divide/1 -> Sum/2
  Abs/1 -> Divide/1
  Discrete-Time Integrator/1 -> z2/1, Divide/2
  Constant/1 -> Divide/3
  Sum/1 -> Discrete-Time Integrator/1

== system VDCHyd2020a/sbHydraulicManipulatorSimscape/sbTiltCylinderAndTiltPiston/sbFrictionForceRS2/sbFrictionRegressorRS2/sbFrictionSwitchingFunctionRS2 ==
  dx2 : Inport
  Abs : Abs
  Constant : Constant  Value=frictionRS2.delta1
  Constant1 : Constant
  Constant2 : Constant
  Discrete-Time Integrator : DiscreteIntegrator  SampleTime=controller.dT  ICPrevOutput=DiscIntNeverNeededParam  ICPrevScaledInput=DiscIntNeverNeededParam
  Divide : Product  Inputs=*/
  Gain : Gain  Gain=10
  Product : Product
  Product1 : Product  Inputs=3
  Sum : Sum  Inputs=|+-
  Sum1 : Sum  Inputs=|++
  LRS2 : Outport
  wires:
  Gain/1 -> Discrete-Time Integrator/1
  Sum/1 -> Gain/1
  Abs/1 -> Sum/1
  dx2/1 -> Abs/1
  Discrete-Time Integrator/1 -> Product/1, Sum/2
  Constant/1 -> Product/2
  Product/1 -> Product1/1, Product1/3, Product1/2
  Product1/1 -> Sum1/1
  Constant1/1 -> Sum1/2
  Sum1/1 -> Divide/2
  Constant2/1 -> Divide/1
  Divide/1 -> LRS2/1

== system VDCHyd2020a/sbVDCController/sbFormAnalyticQuantities/sbPrismaticSegment2/sbGeomPropPS2/sbDiscreteDerivative ==
  xt2 : Inport
  Add : Sum  Inputs=-+
  Gain6 : Gain  Gain=1/(2*controller.dT)
  Integer Delay : Delay  InitialConditionSource=Input port  InitialCondition=0  SampleTime=controller.dT
      settings: InputPortMap=u0,p4
  xt2Velocity : Outport  PortDimensions=1
  wires:
  xt2/1 -> Integer Delay/1, Integer Delay/2, Add/2
  Gain6/1 -> xt2Velocity/1
  Integer Delay/1 -> Add/1
  Add/1 -> Gain6/1

== system VDCHyd2020a/sbVDCController/sbFormAnalyticQuantities/sbRevoluteSegment1/sbGeomPropRS1/sbLiftPistonStroke ==
  note: Get inputs...
  note: Process data...
  note: Pass to outputs...
  q1 : Inport  Unit=rad  PortDimensions=1
  liftPistonStroke : MATLAB Function  TreatAsAtomicUnit=on
  x1 : Outport  Unit=m  PortDimensions=1
  wires:
  [x1] -> x1/1  "x1"
  liftPistonStroke/1(x1) -> [x1]  "x1"
  [q1] -> liftPistonStroke/1(q1)  "q1"
  q1/1 -> [q1]  "q1"

== system VDCHyd2020a/sbVDCController/sbFormAnalyticQuantities/sbRevoluteSegment1/sbGeomPropRS1/sbLiftPistonVelocity ==
  note: Get inputs...
  note: Process data...
  note: Pass to output...
  dq1 : Inport
  x1 : Inport  Port=2
  q1 : Inport  Port=3
  liftPistonVelocity : MATLAB Function  TreatAsAtomicUnit=on
  dx1 : Outport
  wires:
  [dx1] -> dx1/1  "dx1"
  liftPistonVelocity/1(dx1) -> [dx1]  "dx1"
  [q1] -> liftPistonVelocity/3(q1)  "q1"
  q1/1 -> [q1]  "q1"
  [x1] -> liftPistonVelocity/2(x1)  "x1"
  x1/1 -> [x1]  "x1"
  [dq1] -> liftPistonVelocity/1(dq1)  "dq1"
  dq1/1 -> [dq1]  "dq1"

== system VDCHyd2020a/sbVDCController/sbFormAnalyticQuantities/sbRevoluteSegment1/sbGeomPropRS1/sbq11AngleValue ==
  note: Get inputs...
  note: Process data...
  note: Pass to outputs...
  x1 : Inport
  q11AngleValue : MATLAB Function  TreatAsAtomicUnit=on
  q11 : Outport
  wires:
  [q11] -> q11/1  "q11"
  q11AngleValue/1(q11) -> [q11]  "q11"
  [x1] -> q11AngleValue/1(x1)  "x1"
  x1/1 -> [x1]  "x1"

== system VDCHyd2020a/sbVDCController/sbFormAnalyticQuantities/sbRevoluteSegment1/sbGeomPropRS1/sbq11AngleVelocity ==
  note: Get inputs...
  note: Process data...
  note: Pass to outputs...
  x1 : Inport
  q11 : Inport  Port=2
  dx1 : Inport  Port=3
  q11AngleRate : MATLAB Function  TreatAsAtomicUnit=on
  dq11 : Outport
  wires:
  [dq11] -> dq11/1  "dq11"
  q11AngleRate/1(dq11) -> [dq11]  "dq11"
  [dx1] -> q11AngleRate/3(dx1)  "dx1"
  [q11] -> q11AngleRate/2(q11)  "q11"
  [x1] -> q11AngleRate/1(x1)  "x1"
  dx1/1 -> [dx1]  "dx1"
  q11/1 -> [q11]  "q11"
  x1/1 -> [x1]  "x1"

== system VDCHyd2020a/sbVDCController/sbFormAnalyticQuantities/sbRevoluteSegment1/sbGeomPropRS1/sbq12AngleRate ==
  note: Get inputs...
  note: Pass to outputs...
  note: Process data...
  x1 : Inport
  q12 : Inport  Port=2
  dx1 : Inport  Port=3
  q12AngleRate : MATLAB Function  TreatAsAtomicUnit=on
  dq12 : Outport
  wires:
  [dx1] -> q12AngleRate/3(dx1)  "dx1"
  [x1] -> q12AngleRate/1(x1)  "x1"
  [q12] -> q12AngleRate/2(q12)  "q12"
  x1/1 -> [x1]  "x1"
  q12AngleRate/1(dq12) -> [dq12]  "dq12"
  [dq12] -> dq12/1  "dq12"
  q12/1 -> [q12]  "q12"
  dx1/1 -> [dx1]  "dx1"

== system VDCHyd2020a/sbVDCController/sbFormAnalyticQuantities/sbRevoluteSegment1/sbGeomPropRS1/sbq12AngleValue ==
  note: Get inputs...
  note: Process data...
  note: Pass to outputs...
  x1 : Inport
  q12AngleValue : MATLAB Function  TreatAsAtomicUnit=on
  q12 : Outport
  wires:
  [q12] -> q12/1  "q12"
  q12AngleValue/1(q12) -> [q12]  "q12"
  [x1] -> q12AngleValue/1(x1)  "x1"
  x1/1 -> [x1]  "x1"

== system VDCHyd2020a/sbVDCController/sbFormAnalyticQuantities/sbRevoluteSegment1/sbGeomPropRS1/sbq1AngleRate ==
  note: Get inputs...
  note: Process data...
  note: Pass to outputs...
  q1 : Inport
  sbDiscreteDerivative : Subsystem
  dq1 : Outport
  wires:
  sbDiscreteDerivative/1(q1AngleRate) -> [dq1]  "dq1"
  [dq1] -> dq1/1  "dq1"
  [q1] -> sbDiscreteDerivative/1(q1Angle)  "q1"
  q1/1 -> [q1]  "q1"

== system VDCHyd2020a/sbVDCController/sbFormAnalyticQuantities/sbRevoluteSegment1/sbGeomPropRS1req/sbRequiredLiftPistonVelocity ==
  note: Pass to output...
  note: Process data...
  note: Get inputs...
  dq1r : Inport
  x1 : Inport  Port=2
  q1 : Inport  Port=3
  requiredLiftPistonVelocity : MATLAB Function  TreatAsAtomicUnit=on
  dx1r : Outport
  wires:
  dq1r/1 -> [dq1r]  "dq1r"
  [dq1r] -> requiredLiftPistonVelocity/1(dq1r)  "dq1r"
  x1/1 -> [x1]  "x1"
  [x1] -> requiredLiftPistonVelocity/2(x1)  "x1"
  q1/1 -> [q1]  "q1"
  [q1] -> requiredLiftPistonVelocity/3(q1)  "q1"
  requiredLiftPistonVelocity/1(dx1r) -> [dx1r]  "dx1r"
  [dx1r] -> dx1r/1  "dx1r"

== system VDCHyd2020a/sbVDCController/sbFormAnalyticQuantities/sbRevoluteSegment1/sbGeomPropRS1req/sbRequiredq11AngleRate ==
  note: Pass to outputs...
  note: Process data...
  note: Get inputs...
  x1 : Inport
  q11 : Inport  Port=2
  dx1r : Inport  Port=3
  requiredq11AngleRate : MATLAB Function  TreatAsAtomicUnit=on
  dq11r : Outport
  wires:
  x1/1 -> [x1]  "x1"
  q11/1 -> [q11]  "q11"
  dx1r/1 -> [dx1r]  "dx1r"
  [x1] -> requiredq11AngleRate/1(x1)  "x1"
  [q11] -> requiredq11AngleRate/2(q11)  "q11"
  [dx1r] -> requiredq11AngleRate/3(dx1r)  "dx1r"
  requiredq11AngleRate/1(dq11r) -> [dq11r]  "dq11r"
  [dq11r] -> dq11r/1  "dq11r"

== system VDCHyd2020a/sbVDCController/sbFormAnalyticQuantities/sbRevoluteSegment1/sbGeomPropRS1req/sbRequiredq12AngleRate ==
  note: Process data...
  note: Pass to outputs...
  note: Get inputs...
  x1 : Inport
  q12 : Inport  Port=2
  dx1r : Inport  Port=3
  requiredq12AngleRate : MATLAB Function  TreatAsAtomicUnit=on
  dq12r : Outport
  wires:
  dx1r/1 -> [dx1r]  "dx1r"
  q12/1 -> [q12]  "q12"
  [dq12r] -> dq12r/1  "dq12r"
  requiredq12AngleRate/1(dq12r) -> [dq12r]  "dq12r"
  x1/1 -> [x1]  "x1"
  [q12] -> requiredq12AngleRate/2(q12)  "q12"
  [x1] -> requiredq12AngleRate/1(x1)  "x1"
  [dx1r] -> requiredq12AngleRate/3(dx1r)  "dx1r"

== system VDCHyd2020a/sbVDCController/sbFormAnalyticQuantities/sbRevoluteSegment2/sbGeomPropRS2/sbTiltPistonStroke ==
  note: Pass to outputs...
  note: Get inputs...
  note: Derive the tilt piston stroke from q2-angle value...
  note: Process data...
  q2 : Inport
  tiltPistonStroke : MATLAB Function  TreatAsAtomicUnit=on
  x2 : Outport
  wires:
  q2/1 -> [q2]  "q2"
  [x2] -> x2/1  "x2"
  tiltPistonStroke/1(x2) -> [x2]  "x2"
  [q2] -> tiltPistonStroke/1(q2)  "q2"

== system VDCHyd2020a/sbVDCController/sbFormAnalyticQuantities/sbRevoluteSegment2/sbGeomPropRS2/sbTiltPistonVelocity ==
  note: Get inputs...
  note: Process data...
  note: Pass to output...
  dq2 : Inport
  x2 : Inport  Port=2
  q2 : Inport  Port=3
  tiltPistonVelocity : MATLAB Function  TreatAsAtomicUnit=on
  dx2 : Outport
  wires:
  tiltPistonVelocity/1(dx2) -> [dx2]  "dx2"
  [dx2] -> dx2/1  "dx2"
  [q2] -> tiltPistonVelocity/3(q2)  "q2"
  q2/1 -> [q2]  "q2"
  [x2] -> tiltPistonVelocity/2(x2)  "x2"
  x2/1 -> [x2]  "x2"
  [dq2] -> tiltPistonVelocity/1(dq2)  "dq2"
  dq2/1 -> [dq2]  "dq2"

== system VDCHyd2020a/sbVDCController/sbFormAnalyticQuantities/sbRevoluteSegment2/sbGeomPropRS2/sbq21AngleRate ==
  note: Get inputs...
  note: Process data...
  note: Pass to outputs...
  x2 : Inport
  q21 : Inport  Port=2
  dx2 : Inport  Port=3
  q21AngleRate : MATLAB Function  TreatAsAtomicUnit=on
  dq21 : Outport
  wires:
  [q21] -> q21AngleRate/2(q21)  "q21"
  [dx2] -> q21AngleRate/3(dx2)  "dx2"
  [dq21] -> dq21/1  "dq21"
  q21AngleRate/1(dq21) -> [dq21]  "dq21"
  [x2] -> q21AngleRate/1(x2)  "x2"
  dx2/1 -> [dx2]  "dx2"
  q21/1 -> [q21]  "q21"
  x2/1 -> [x2]  "x2"

== system VDCHyd2020a/sbVDCController/sbFormAnalyticQuantities/sbRevoluteSegment2/sbGeomPropRS2/sbq21AngleValue ==
  note: Get inputs...
  note: Process data...
  note: Pass to outputs...
  x2 : Inport
  q21AngleValue : MATLAB Function  TreatAsAtomicUnit=on
  q21 : Outport
  wires:
  q21AngleValue/1(q21) -> [q21]  "q21"
  [x2] -> q21AngleValue/1(x2)  "x2"
  [q21] -> q21/1  "q21"
  x2/1 -> [x2]  "x2"

== system VDCHyd2020a/sbVDCController/sbFormAnalyticQuantities/sbRevoluteSegment2/sbGeomPropRS2/sbq22AngleRate ==
  note: Get inputs...
  note: Pass to outputs...
  note: Process data...
  x2 : Inport
  q22 : Inport  Port=2
  dx2 : Inport  Port=3
  q22AngleRate : MATLAB Function  TreatAsAtomicUnit=on
  dq22 : Outport
  wires:
  [x2] -> q22AngleRate/1(x2)  "x2"
  x2/1 -> [x2]  "x2"
  q22AngleRate/1(dq22) -> [dq22]  "dq22"
  [dq22] -> dq22/1  "dq22"
  q22/1 -> [q22]  "q22"
  dx2/1 -> [dx2]  "dx2"
  [q22] -> q22AngleRate/2(q22)  "q22"
  [dx2] -> q22AngleRate/3(dx2)  "dx2"

== system VDCHyd2020a/sbVDCController/sbFormAnalyticQuantities/sbRevoluteSegment2/sbGeomPropRS2/sbq22AngleValue ==
  note: Pass to outputs...
  note: Process data...
  note: Get inputs...
  x2 : Inport
  q22AngleValue : MATLAB Function  TreatAsAtomicUnit=on
  q22 : Outport
  wires:
  x2/1 -> [x2]  "x2"
  [x2] -> q22AngleValue/1(x2)  "x2"
  q22AngleValue/1(q22) -> [q22]  "q22"
  [q22] -> q22/1  "q22"

== system VDCHyd2020a/sbVDCController/sbFormAnalyticQuantities/sbRevoluteSegment2/sbGeomPropRS2/sbq2AngleRate ==
  note: Get inputs...
  note: Process data...
  note: Pass to outputs...
  q2 : Inport
  sbDiscreteDerivative : Subsystem
  dq2 : Outport
  wires:
  sbDiscreteDerivative/1(q2AngleRate) -> [dq2]  "dq2"
  [dq2] -> dq2/1  "dq2"
  [q2] -> sbDiscreteDerivative/1(q2Angle)  "q2"
  q2/1 -> [q2]  "q2"

== system VDCHyd2020a/sbVDCController/sbFormAnalyticQuantities/sbRevoluteSegment2/sbGeomPropRS2req/sbRequiredTiltPistonVelocity ==
  note: Pass to output...
  note: Process data...
  note: Get inputs...
  dq2r : Inport
  x2 : Inport  Port=2
  q2 : Inport  Port=3
  requiredTiltPistonVelocity : MATLAB Function  TreatAsAtomicUnit=on
  dx2r : Outport
  wires:
  dq2r/1 -> [dq2r]  "dq2r"
  [dq2r] -> requiredTiltPistonVelocity/1(dq2r)  "dq2r"
  x2/1 -> [x2]  "x2"
  [x2] -> requiredTiltPistonVelocity/2(x2)  "x2"
  q2/1 -> [q2]  "q2"
  [q2] -> requiredTiltPistonVelocity/3(q2)  "q2"
  [dx2r] -> dx2r/1  "dx2r"
  requiredTiltPistonVelocity/1(dx2r) -> [dx2r]  "dx2r"

== system VDCHyd2020a/sbVDCController/sbFormAnalyticQuantities/sbRevoluteSegment2/sbGeomPropRS2req/sbRequiredq21AngleRate ==
  note: Pass to outputs...
  note: Process data...
  note: Get inputs...
  x2 : Inport
  q21 : Inport  Port=2
  dx2r : Inport  Port=3
  requiredq21AngleRate : MATLAB Function  TreatAsAtomicUnit=on
  dq21r : Outport
  wires:
  x2/1 -> [x2]  "x2"
  q21/1 -> [q21]  "q21"
  dx2r/1 -> [dx2r]  "dx2r"
  [x2] -> requiredq21AngleRate/1(x2)  "x2"
  requiredq21AngleRate/1(dq21r) -> [dq21r]  "dq21r"
  [dq21r] -> dq21r/1  "dq21r"
  [dx2r] -> requiredq21AngleRate/3(dx2r)  "dx2r"
  [q21] -> requiredq21AngleRate/2(q21)  "q21"

== system VDCHyd2020a/sbVDCController/sbFormAnalyticQuantities/sbRevoluteSegment2/sbGeomPropRS2req/sbRequiredq22AngleRate ==
  note: Process data...
  note: Pass to outputs...
  note: Get inputs...
  x2 : Inport
  q22 : Inport  Port=2
  dx2r : Inport  Port=3
  requiredq22AngleRate : MATLAB Function  TreatAsAtomicUnit=on
  dq22r : Outport
  wires:
  dx2r/1 -> [dx2r]  "dx2r"
  q22/1 -> [q22]  "q22"
  [dq22r] -> dq22r/1  "dq22r"
  requiredq22AngleRate/1(dq22r) -> [dq22r]  "dq22r"
  x2/1 -> [x2]  "x2"
  [x2] -> requiredq22AngleRate/1(x2)  "x2"
  [dx2r] -> requiredq22AngleRate/3(dx2r)  "dx2r"
  [q22] -> requiredq22AngleRate/2(q22)  "q22"

== system VDCHyd2020a/sbVDCController/sbFormTotalRequiredForces/sbTotalRequiredForcesPS2/sbFilteredVelocityDerivativeB52/sbDiscreteDerivative1 ==
  u : Inport
  Add : Sum  Inputs=-+
  Gain6 : Gain  Gain=1/(2*controller.dT)
  Integer Delay : Delay  InitialConditionSource=Input port  InitialCondition=0  SampleTime=controller.dT
      settings: InputPortMap=u0,p4
  du/dt : Outport  PortDimensions=1
  wires:
  Add/1 -> Gain6/1
  u/1 -> Integer Delay/1, Integer Delay/2, Add/2
  Integer Delay/1 -> Add/1
  Gain6/1 -> du/dt/1

== system VDCHyd2020a/sbVDCController/sbFormTotalRequiredForces/sbTotalRequiredForcesPS2/sbFilteredVelocityDerivativeB52/sbDiscreteDerivative2 ==
  u : Inport
  Add : Sum  Inputs=-+
  Gain6 : Gain  Gain=1/(2*controller.dT)
  Integer Delay : Delay  InitialConditionSource=Input port  InitialCondition=0  SampleTime=controller.dT
      settings: InputPortMap=u0,p4
  du/dt : Outport  PortDimensions=1
  wires:
  u/1 -> Integer Delay/1, Integer Delay/2, Add/2
  Integer Delay/1 -> Add/1
  Add/1 -> Gain6/1
  Gain6/1 -> du/dt/1

== system VDCHyd2020a/sbVDCController/sbFormTotalRequiredForces/sbTotalRequiredForcesPS2/sbFilteredVelocityDerivativeB52/sbDiscreteDerivative3 ==
  u : Inport
  Add : Sum  Inputs=-+
  Gain6 : Gain  Gain=1/(2*controller.dT)
  Integer Delay : Delay  InitialConditionSource=Input port  InitialCondition=0  SampleTime=controller.dT
      settings: InputPortMap=u0,p4
  du/dt : Outport  PortDimensions=1
  wires:
  Add/1 -> Gain6/1
  Integer Delay/1 -> Add/1
  u/1 -> Integer Delay/1, Integer Delay/2, Add/2
  Gain6/1 -> du/dt/1

== system VDCHyd2020a/sbVDCController/sbFormTotalRequiredForces/sbTotalRequiredForcesPS2/sbFilteredVelocityDerivativeB52/sbDiscreteDerivative4 ==
  u : Inport
  Add : Sum  Inputs=-+
  Gain6 : Gain  Gain=1/(2*controller.dT)
  Integer Delay : Delay  InitialConditionSource=Input port  InitialCondition=0  SampleTime=controller.dT
      settings: InputPortMap=u0,p4
  du/dt : Outport  PortDimensions=1
  wires:
  Add/1 -> Gain6/1
  Integer Delay/1 -> Add/1
  u/1 -> Integer Delay/1, Integer Delay/2, Add/2
  Gain6/1 -> du/dt/1

== system VDCHyd2020a/sbVDCController/sbFormTotalRequiredForces/sbTotalRequiredForcesPS2/sbFilteredVelocityDerivativeB52/sbDiscreteDerivative5 ==
  u : Inport
  Add : Sum  Inputs=-+
  Gain6 : Gain  Gain=1/(2*controller.dT)
  Integer Delay : Delay  InitialConditionSource=Input port  InitialCondition=0  SampleTime=controller.dT
      settings: InputPortMap=u0,p4
  du/dt : Outport  PortDimensions=1
  wires:
  Add/1 -> Gain6/1
  Integer Delay/1 -> Add/1
  u/1 -> Integer Delay/1, Integer Delay/2, Add/2
  Gain6/1 -> du/dt/1

== system VDCHyd2020a/sbVDCController/sbFormTotalRequiredForces/sbTotalRequiredForcesPS2/sbFilteredVelocityDerivativeB52/sbDiscreteDerivative6 ==
  u : Inport
  Add : Sum  Inputs=-+
  Gain6 : Gain  Gain=1/(2*controller.dT)
  Integer Delay : Delay  InitialConditionSource=Input port  InitialCondition=0  SampleTime=controller.dT
      settings: InputPortMap=u0,p4
  du/dt : Outport  PortDimensions=1
  wires:
  Add/1 -> Gain6/1
  Integer Delay/1 -> Add/1
  u/1 -> Integer Delay/1, Integer Delay/2, Add/2
  Gain6/1 -> du/dt/1
